simulink model "E2_1_Effort"  (R2022a)
settings: Solver=VariableStepAuto  StartTime=0.0  StopTime=10.0  RelTol=1e-3
settings Model: Creator=Reza  LastModifiedBy=Reza

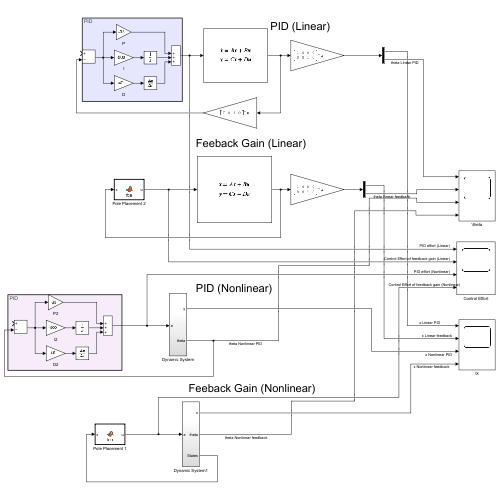
[thumbnail: Simulink's stored preview of the top-level diagram]
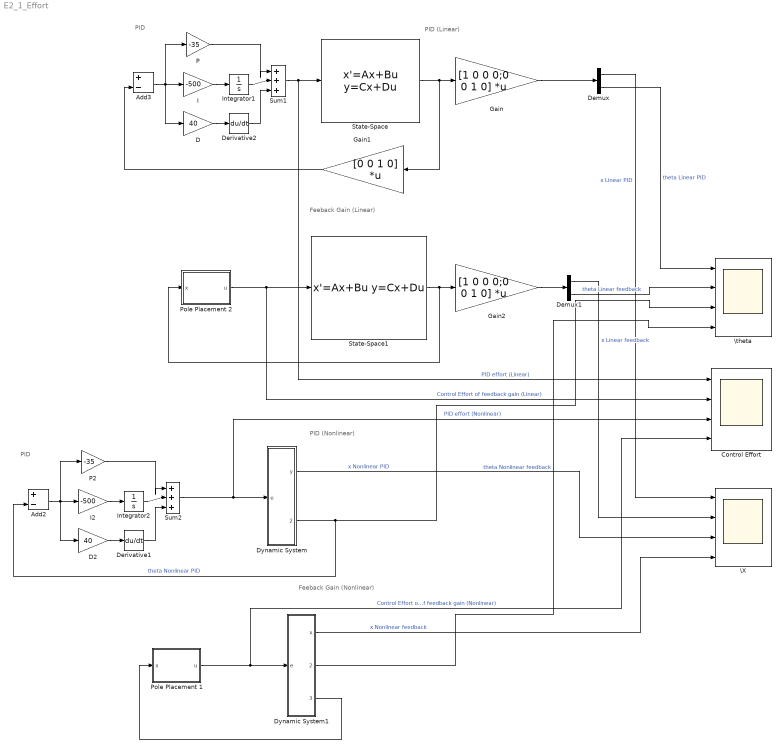
== system E2_1_Effort ==
  note: PID
  note: PID
  note: PID (Nonlinear)
  note: Feeback Gain (Nonlinear)
  note: Feeback Gain (Linear)
  note: PID (Linear)
  Add2 : Sum  Inputs=+-
  Add3 : Sum  Inputs=+-
  Control Effort : Scope  NumInputPorts=4
  D : Gain  Gain=40
  D2 : Gain  Gain=40
  Demux : Demux  Outputs=2
  Demux1 : Demux  Outputs=2
  Derivative1 : Derivative
  Derivative2 : Derivative
  Dynamic System : Subsystem
  Dynamic System1 : Subsystem
  Gain : Gain  Gain=[1 0 0 0;0 0 1 0]  Multiplication=Matrix(K*u)
  Gain1 : Gain  Gain=[0 0 1 0]  Multiplication=Matrix(K*u)
  Gain2 : Gain  Gain=[1 0 0 0;0 0 1 0]  Multiplication=Matrix(K*u)
  I : Gain  Gain=-500
  I2 : Gain  Gain=-500
  Integrator1 : Integrator
  Integrator2 : Integrator
  P : Gain  Gain=-35
  P2 : Gain  Gain=-35
  Pole Placement 1 : MATLAB Function  TreatAsAtomicUnit=on
  Pole Placement 2 : MATLAB Function  TreatAsAtomicUnit=on
  State-Space : StateSpace  A=[0 1 0 0;0 -25 -0.98 0;0 0 0 1;0 25 10.78 0]  B=[0;0.5;0;-0.5]  C=eye(4)  D=[0;0;0;0]  InitialCondition=[0;0;10*pi/180;0]
  State-Space1 : StateSpace  A=[0 1 0 0;0 -25 -0.98 0;0 0 0 1;0 25 10.78 0]  B=[0;0.5;0;-0.5]  C=eye(4)  D=[0;0;0;0]  InitialCondition=[0;0;10*pi/180;0]
  Sum1 : Sum  Inputs=|+++
  Sum2 : Sum  Inputs=|+++
  \X : Scope  NumInputPorts=4
  \theta : Scope  NumInputPorts=4
  wires:
  State-Space/1 -> Gain1/1, Gain/1
  Gain1/1 -> Add3/2
  State-Space1/1 -> Pole Placement 2/1(x), Gain2/1
  Pole Placement 2/1(u) -> Control Effort/2, State-Space1/1  "Control Effort of feedback gain (Linear)"
  Gain/1 -> Demux/1
  Gain2/1 -> Demux1/1
  Sum1/1 -> State-Space/1, Control Effort/1  "PID effort (Linear)"
  Dynamic System1/3(States) -> Pole Placement 1/1(x)
  Sum2/1 -> Control Effort/3, Dynamic System/1(e)  "PID effort (Nonlinear)"
  Pole Placement 1/1(u) -> Control Effort/4, Dynamic System1/1(e)  "Control Effort of feedback gain (Nonlinear)"
  Dynamic System/2(theta) -> \theta/3, Add2/2  "theta Nonlinear PID"
  Dynamic System1/2(theta) -> \theta/4  "theta Nonlinear feedback"
  P/1 -> Sum1/1
  Add3/1 -> D/1, I/1, P/1
  I/1 -> Integrator1/1
  D/1 -> Derivative2/1
  Derivative2/1 -> Sum1/3
  Integrator1/1 -> Sum1/2
  Derivative1/1 -> Sum2/3
  I2/1 -> Integrator2/1
  P2/1 -> Sum2/1
  D2/1 -> Derivative1/1
  Add2/1 -> D2/1, I2/1, P2/1
  Integrator2/1 -> Sum2/2
  Dynamic System1/1(x) -> \X/4  "x Nonlinear feedback"
  Dynamic System/1(y) -> \X/3  "x Nonlinear PID"
  Demux/2 -> \theta/1  "theta Linear PID"
  Demux1/2 -> \theta/2  "theta Linear feedback"
  Demux/1 -> \X/1  "x Linear PID"
  Demux1/1 -> \X/2  "x Linear feedback"

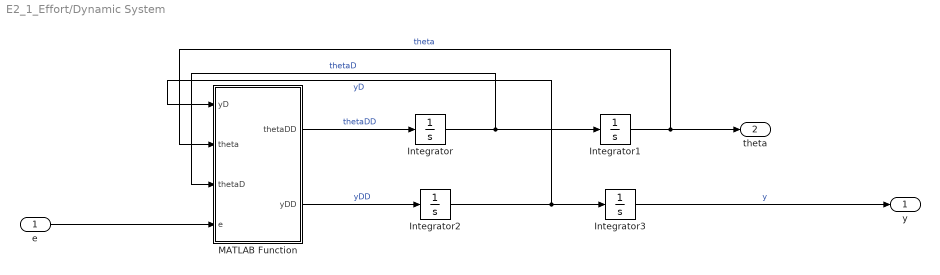
== system E2_1_Effort/Dynamic System ==
  e : Inport
  Integrator : Integrator
  Integrator1 : Integrator  InitialCondition=10*pi/180
  Integrator2 : Integrator
  Integrator3 : Integrator
  MATLAB Function : MATLAB Function  TreatAsAtomicUnit=on
  y : Outport
  theta : Outport  Port=2
  wires:
  Integrator/1 -> MATLAB Function/3(thetaD), Integrator1/1  "thetaD"
  Integrator1/1 -> theta/1, MATLAB Function/2(theta)  "theta"
  MATLAB Function/1(thetaDD) -> Integrator/1  "thetaDD"
  Integrator2/1 -> MATLAB Function/1(yD), Integrator3/1  "yD"
  e/1 -> MATLAB Function/4(e)
  MATLAB Function/2(yDD) -> Integrator2/1  "yDD"
  Integrator3/1 -> y/1  "y"

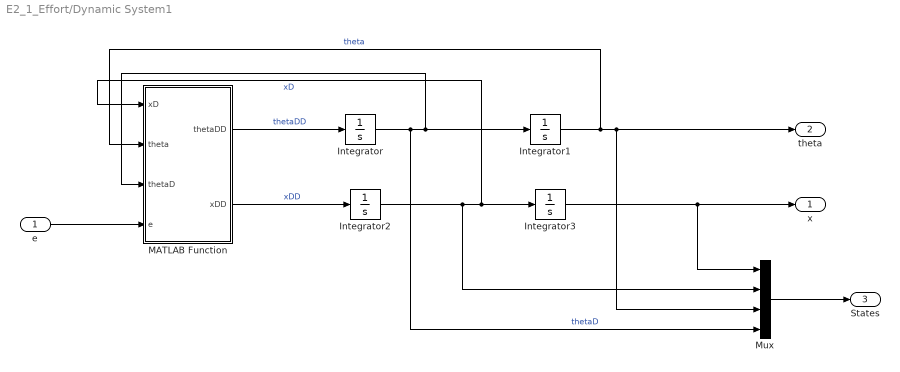
== system E2_1_Effort/Dynamic System1 ==
  e : Inport
  Integrator : Integrator
  Integrator1 : Integrator  InitialCondition=10*pi/180
  Integrator2 : Integrator
  Integrator3 : Integrator
  MATLAB Function : MATLAB Function  TreatAsAtomicUnit=on
  Mux : Mux
  x : Outport
  theta : Outport  Port=2
  States : Outport  Port=3
  wires:
  MATLAB Function/2(xDD) -> Integrator2/1  "xDD"
  e/1 -> MATLAB Function/4(e)
  Integrator2/1 -> Mux/2, Integrator3/1, MATLAB Function/1(xD)  "xD"
  MATLAB Function/1(thetaDD) -> Integrator/1  "thetaDD"
  Integrator1/1 -> MATLAB Function/2(theta), Mux/3, theta/1  "theta"
  Integrator/1 -> Mux/4, Integrator1/1, MATLAB Function/3(thetaD)  "thetaD"
  Mux/1 -> States/1
  Integrator3/1 -> Mux/1, x/1

== matlab function E2_1_Effort/Dynamic System1/MATLAB Function ==
  data: thetaDD output; xD input; theta input; thetaD input; e input; xDD output
function [thetaDD,xDD] = fcn(xD,theta,thetaD,e)
k = 1 ; m = 0.1 ; M = 1 ; R = 100 ; r = 0.02 ; l = 1 ; g = 9.8 ; 
thetaDD = (m*l*sin(theta)*thetaD^2 - k^2/(R*r^2)*xD + k/(R*r)*e + (M+m)*(tan(theta)*xD*thetaD + g*tan(theta)))/(m*l*cos(theta)-(M+m)/cos(theta)) ; 
xDD = tan(theta)*xD*thetaD + g*tan(theta) - thetaDD/cos(theta) ;

== matlab function E2_1_Effort/Dynamic System/MATLAB Function ==
  data: thetaDD output; yD input; theta input; thetaD input; e input; yDD output
function [thetaDD,yDD] = fcn(yD,theta,thetaD,e)
k = 1 ; m = 0.1 ; M = 1 ; R = 100 ; r = 0.02 ; l = 1 ; g = 9.8 ; 
thetaDD = (m*l*sin(theta)*thetaD^2 - k^2/(R*r^2)*yD + k/(R*r)*e + (M+m)*(tan(theta)*yD*thetaD + g*tan(theta)))/(m*l*cos(theta)-(M+m)/cos(theta)) ; 
yDD = tan(theta)*yD*thetaD + g*tan(theta) - thetaDD/cos(theta) ;

== matlab function E2_1_Effort/Pole Placement 2 ==
  data: x input; u output
function u = fcn(x)
K = [-326.5306 , -226.3265 , -812.0906 , -242.3265] ; 
u = -K*x ;

== matlab function E2_1_Effort/Pole Placement 1 ==
  data: x input; u output
function u = fcn(x)
K = [-326.5306 , -226.3265 , -812.0906 , -242.3265] ; 
u = -K*x ;
